simulink model "OFDMTxRx2211221"  (R2017b)
settings: Solver=VariableStepAuto  StartTime=0.0  StopTime=10  RelTol=1e-3
InitFcn:
  | Ts = 1e-6;
  | simParams.Ts = Ts;
  | simParams.TsTx = Ts;
  | simParams.TsRx = Ts;
  | simParams.nFFT = 1024;
  | simParams.lengthCP = 128;
  | nFFT = simParams.nFFT;
  | simParams.NSubcarriers = 398;
  | simParams.windowing = 16;
undefined symbols (not defined in the file): fft_size, i
libraries: hdlsllib x35, simulink x28, simulink_need_slupdate x17, dspmathops x5, dspxfrm3 x3, dspsigops x2, commdigbbndam3 x1, commrflib2 x1, commseqgen3 x1
(part 2 of 3)

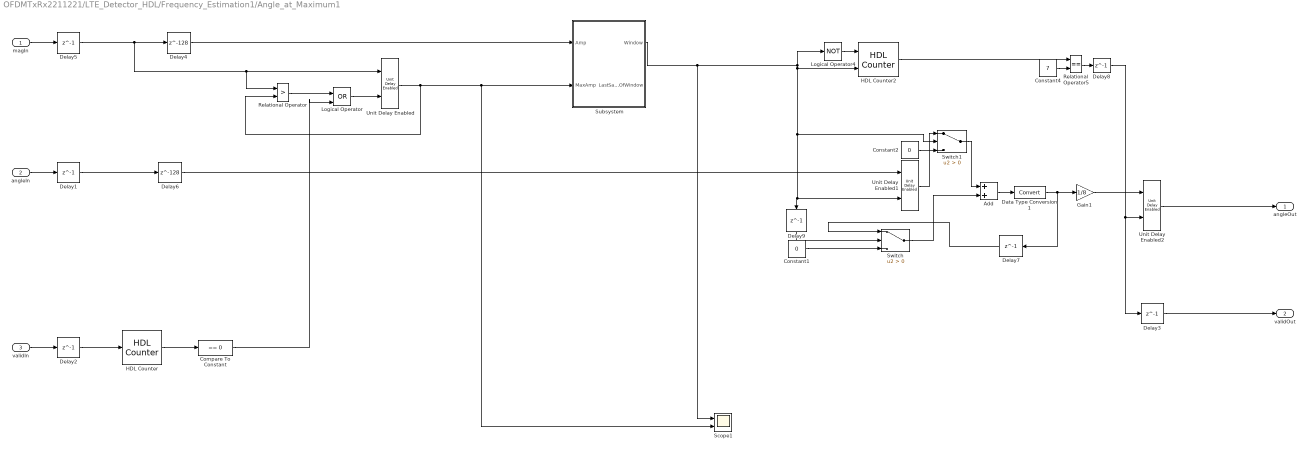
== system OFDMTxRx2211221/LTE_Detector_HDL/Frequency_Estimation1/Angle_at_Maximum1 ==
  magIn : Inport
  angleIn : Inport  Port=2
  validIn : Inport  Port=3
  Add : Sum
  Compare To Constant : simulink/Logic and Bit Operations/Compare To Constant  relop===  const=0  OutDataTypeStr=boolean
  Constant1 : Constant  Value=0
  Constant2 : Constant  Value=0
  Constant4 : Constant  Value=7
  Data Type Conversion1 : DataTypeConversion
  Delay{1..3,5,7..9} (7 alike) : Delay  DelayLength=1  InitialCondition=0  UseCircularBuffer=on
  Delay4 : Delay  DelayLength=128  InitialCondition=0  UseCircularBuffer=on
  Delay6 : Delay  DelayLength=128  InitialCondition=0  UseCircularBuffer=on
  Gain1 : Gain  Gain=1/8
  HDL Counter : hdlsllib/Sources/HDL Counter  CountType=Count limited  CountInit=0  CountStep=1  CountMax=1152  CountFromType=Initial value  CountFrom=0  CountResetPort=off  CountLoadPort=off  CountEnbPort=on  CountDirPort=off  CountDataType=Unsigned  CountWordLen=11  CountFracLen=0  CountSampTime=1
      settings: SourceProductBaseCode=HD
  HDL Counter2 : hdlsllib/Sources/HDL Counter  CountType=Count limited  CountInit=0  CountStep=1  CountMax=7  CountFromType=Initial value  CountFrom=0  CountResetPort=on  CountLoadPort=off  CountEnbPort=on  CountDirPort=off  CountDataType=Unsigned  CountWordLen=3  CountFracLen=0  CountSampTime=1
      settings: SourceProductBaseCode=HD
  Logical Operator : Logic  Operator=OR  IconShape=distinctive  AllPortsSameDT=off  OutDataTypeStr=boolean
  Logical Operator4 : Logic  Operator=NOT  IconShape=distinctive  AllPortsSameDT=off  OutDataTypeStr=boolean
  Relational Operator : RelationalOperator  Operator=>  OutDataTypeStr=boolean  RndMeth=Nearest
  Relational Operator5 : RelationalOperator  Operator===  OutDataTypeStr=boolean  RndMeth=Nearest
  Scope1 : Scope  NumInputPorts=2
  Subsystem : Subsystem
  Switch : Switch  Criteria=u2 > Threshold
  Switch1 : Switch  Criteria=u2 > Threshold
  Unit Delay Enabled : simulink_need_slupdate/Unit Delay Enabled  vinit=0.0  tsamp=-1
      settings: SourceProductName=Simulink  SourceProductBaseCode=SL
  Unit Delay Enabled1 : simulink_need_slupdate/Unit Delay Enabled  vinit=0.0  tsamp=-1
      settings: SourceProductName=Simulink  SourceProductBaseCode=SL
  Unit Delay Enabled2 : simulink_need_slupdate/Unit Delay Enabled  vinit=0.0  tsamp=-1
      settings: SourceProductName=Simulink  SourceProductBaseCode=SL
  angleOut : Outport
  validOut : Outport  Port=2
  wires:
  Delay4/1 -> Subsystem/1(Amp)
  Unit Delay Enabled1/1 -> Switch1/1
  Unit Delay Enabled2/1 -> angleOut/1
  Compare To Constant/1 -> Logical Operator/2
  Logical Operator/1 -> Unit Delay Enabled/2
  Constant1/1 -> Switch/3
  Delay7/1 -> Switch/1
  Delay3/1 -> validOut/1
  Constant2/1 -> Switch1/3
  Gain1/1 -> Unit Delay Enabled2/1
  Subsystem/1(Window) -> Scope1/1, Switch1/2, Delay9/1, Unit Delay Enabled1/2, HDL Counter2/2, Logical Operator4/1
  Delay9/1 -> Switch/2
  Unit Delay Enabled/1 -> Scope1/2, Subsystem/2(MaxAmp), Relational Operator/2
  Data Type Conversion1/1 -> Delay7/1, Gain1/1
  Logical Operator4/1 -> HDL Counter2/1
  Switch1/1 -> Add/1
  Add/1 -> Data Type Conversion1/1
  Relational Operator5/1 -> Delay8/1
  Delay2/1 -> HDL Counter/1
  HDL Counter2/1 -> Relational Operator5/1
  Constant4/1 -> Relational Operator5/2
  Delay8/1 -> Unit Delay Enabled2/2, Delay3/1
  Delay6/1 -> Unit Delay Enabled1/1
  Delay5/1 -> Relational Operator/1, Unit Delay Enabled/1, Delay4/1
  Delay1/1 -> Delay6/1
  validIn/1 -> Delay2/1
  Relational Operator/1 -> Logical Operator/1
  angleIn/1 -> Delay1/1
  HDL Counter/1 -> Compare To Constant/1
  magIn/1 -> Delay5/1
  Switch/1 -> Add/2

== system OFDMTxRx2211221/LTE_Detector_HDL/Frequency_Estimation1/Cyclic_Prefix_Correlator ==
  dataIn : Inport
  Delay1 : Delay  DelayLength=1  InitialCondition=0  UseCircularBuffer=on
  Delay2 : Delay  DelayLength=1024  InitialCondition=0
  Delay3 : Delay  DelayLength=1  InitialCondition=0  UseCircularBuffer=on
  Delay5 : Delay  DelayLength=1  InitialCondition=0  UseCircularBuffer=on
  Moving_Average : Subsystem
  Product : Product  OutDataTypeStr=fixdt(1,24,23)  RndMeth=Round
  Slot_Average : Subsystem
  complexConj : Math  Operator=conj  SaturateOnIntegerOverflow=on
  corrOut : Outport
  wires:
  Delay3/1 -> Product/2
  Delay2/1 -> complexConj/1
  complexConj/1 -> Delay3/1
  Delay1/1 -> Product/1
  Delay5/1 -> Moving_Average/1(dataIn)
  dataIn/1 -> Delay2/1, Delay1/1
  Product/1 -> Delay5/1
  Moving_Average/1(dataOut) -> Slot_Average/1(dataIn)
  Slot_Average/1(dataOut) -> corrOut/1

== system OFDMTxRx2211221/LTE_Detector_HDL/Frequency_Estimation1/Rect_to_Polar ==
  dataIn : Inport
  Complex to Magnitude-Angle HDL Optimized : dspmathops/Complex to Magnitude-Angle HDL Optimized  NumIterationsSource=Auto  NumIterations=16  OutputFormat=Magnitude and angle  AngleFormat=Normalized  ScaleOutput=on  SimulateUsing=Code generation
      settings: SourceProductName=DSP System Toolbox  SourceProductBaseCode=DS
  Constant : Constant  OutDataTypeStr=boolean  SampleTime=simParams.TsRx
  Delay1 : Delay  InitialCondition=0  UseCircularBuffer=on
  Delay2 : Delay  DelayLength=1  InitialCondition=0  UseCircularBuffer=on
  Delay3 : Delay  DelayLength=1  InitialCondition=0  UseCircularBuffer=on
  Delay4 : Delay  DelayLength=1  InitialCondition=0  UseCircularBuffer=on
  Delay5 : Delay  InitialCondition=0  UseCircularBuffer=on
  Gain : Gain  Gain=0.5  OutDataTypeStr=fixdt(1,27,27)
  Signal Specification1 : SignalSpecification  Dimensions=1
  magOut : Outport
  angleOut : Outport  Port=2
  validOut : Outport  Port=3
  wires:
  Gain/1 -> angleOut/1
  dataIn/1 -> Signal Specification1/1
  Constant/1 -> Delay1/1
  Delay5/1 -> Complex to Magnitude-Angle HDL Optimized/1
  Delay1/1 -> Complex to Magnitude-Angle HDL Optimized/2
  Delay2/1 -> magOut/1
  Delay3/1 -> Gain/1
  Delay4/1 -> validOut/1
  Complex to Magnitude-Angle HDL Optimized/1 -> Delay2/1
  Complex to Magnitude-Angle HDL Optimized/3 -> Delay4/1
  Complex to Magnitude-Angle HDL Optimized/2 -> Delay3/1
  Signal Specification1/1 -> Delay5/1

== system OFDMTxRx2211221/LTE_Detector_HDL/Frequency_Estimation2/Angle_at_Maximum ==
  note: This subsystem records the maximum CP correlation level, and the corresponding phase angle of the result, across windows of time equivalent to 1 slot (960 samples). A counter is used to reset the running max and record the final phase value, which is then passed to the output and qualified by the validOut signal.
  note: Store current mag & angle if mag is greater than previous max mag.
  note: This register stores the current running max magnitude in the current time window
  magIn : Inport
  angleIn : Inport  Port=2
  validIn : Inport  Port=3
  Compare To Constant : simulink/Logic and Bit Operations/Compare To Constant  relop===  const=0  OutDataTypeStr=boolean
  Delay{1..3,5} (4 alike) : Delay  DelayLength=1  InitialCondition=0  UseCircularBuffer=on
  HDL Counter : hdlsllib/Sources/HDL Counter  CountType=Count limited  CountInit=0  CountStep=1  CountMax=1152  CountFromType=Initial value  CountFrom=0  CountResetPort=off  CountLoadPort=off  CountEnbPort=on  CountDirPort=off  CountDataType=Unsigned  CountWordLen=11  CountFracLen=0  CountSampTime=1
      settings: SourceProductBaseCode=HD
  Logical Operator : Logic  Operator=OR  IconShape=distinctive  AllPortsSameDT=off  OutDataTypeStr=boolean
  Relational Operator : RelationalOperator  Operator=>  OutDataTypeStr=boolean  RndMeth=Nearest
  Unit Delay Enabled : simulink_need_slupdate/Unit Delay Enabled  vinit=0.0  tsamp=-1
      settings: SourceProductName=Simulink  SourceProductBaseCode=SL
  Unit Delay Enabled1 : simulink_need_slupdate/Unit Delay Enabled  vinit=0.0  tsamp=-1
      settings: SourceProductName=Simulink  SourceProductBaseCode=SL
  Unit Delay Enabled2 : simulink_need_slupdate/Unit Delay Enabled  vinit=0.0  tsamp=-1
      settings: SourceProductName=Simulink  SourceProductBaseCode=SL
  angleOut : Outport
  validOut : Outport  Port=2
  wires:
  magIn/1 -> Delay5/1
  angleIn/1 -> Delay1/1
  HDL Counter/1 -> Compare To Constant/1
  Compare To Constant/1 -> Unit Delay Enabled2/2, Logical Operator/2, Delay3/1
  Unit Delay Enabled1/1 -> Unit Delay Enabled2/1
  validIn/1 -> Delay2/1
  Delay5/1 -> Relational Operator/1, Unit Delay Enabled/1
  Delay2/1 -> HDL Counter/1
  Unit Delay Enabled2/1 -> angleOut/1
  Delay3/1 -> validOut/1
  Unit Delay Enabled/1 -> Relational Operator/2
  Relational Operator/1 -> Logical Operator/1
  Logical Operator/1 -> Unit Delay Enabled1/2, Unit Delay Enabled/2
  Delay1/1 -> Unit Delay Enabled1/1

== system OFDMTxRx2211221/LTE_Detector_HDL/Frequency_Estimation2/Cyclic_Prefix_Correlator ==
  note: Correlate the signal with itself
      | delayed by the FFT length (128 samples).
  note: Integrate across part of the CP length, which is 9 samples. However we use 8 samples here to optimize for HDL implementation.
  note: Finally average across 7 OFDM symbols, i.e. the number in
      | each slot.
  dataIn : Inport
  Delay1 : Delay  DelayLength=1  InitialCondition=0  UseCircularBuffer=on
  Delay2 : Delay  DelayLength=1024  InitialCondition=0
  Delay3 : Delay  DelayLength=1  InitialCondition=0  UseCircularBuffer=on
  Delay5 : Delay  DelayLength=1  InitialCondition=0  UseCircularBuffer=on
  Moving_Average : Subsystem
  Product : Product  OutDataTypeStr=fixdt(1,24,23)  RndMeth=Round
  Slot_Average : Subsystem
  complexConj : Math  Operator=conj  SaturateOnIntegerOverflow=on
  corrOut : Outport
  wires:
  Product/1 -> Delay5/1
  Delay3/1 -> Product/2
  Delay2/1 -> complexConj/1
  Slot_Average/1(dataOut) -> corrOut/1
  Moving_Average/1(dataOut) -> Slot_Average/1(dataIn)
  complexConj/1 -> Delay3/1
  Delay5/1 -> Moving_Average/1(dataIn)
  Delay1/1 -> Product/1
  dataIn/1 -> Delay2/1, Delay1/1

== system OFDMTxRx2211221/LTE_Detector_HDL/Frequency_Estimation2/Rect_to_Polar ==
  dataIn : Inport
  Complex to Magnitude-Angle HDL Optimized : dspmathops/Complex to Magnitude-Angle HDL Optimized  NumIterationsSource=Auto  NumIterations=16  OutputFormat=Magnitude and angle  AngleFormat=Normalized  ScaleOutput=on  SimulateUsing=Code generation
      settings: SourceProductName=DSP System Toolbox  SourceProductBaseCode=DS
  Constant : Constant  OutDataTypeStr=boolean  SampleTime=simParams.TsRx
  Delay1 : Delay  InitialCondition=0  UseCircularBuffer=on
  Delay2 : Delay  DelayLength=1  InitialCondition=0  UseCircularBuffer=on
  Delay3 : Delay  DelayLength=1  InitialCondition=0  UseCircularBuffer=on
  Delay4 : Delay  DelayLength=1  InitialCondition=0  UseCircularBuffer=on
  Delay5 : Delay  InitialCondition=0  UseCircularBuffer=on
  Gain : Gain  Gain=0.5  OutDataTypeStr=fixdt(1,27,27)
  Signal Specification1 : SignalSpecification  Dimensions=1
  magOut : Outport
  angleOut : Outport  Port=2
  validOut : Outport  Port=3
  wires:
  Gain/1 -> angleOut/1
  dataIn/1 -> Signal Specification1/1
  Constant/1 -> Delay1/1
  Delay5/1 -> Complex to Magnitude-Angle HDL Optimized/1
  Delay1/1 -> Complex to Magnitude-Angle HDL Optimized/2
  Delay2/1 -> magOut/1
  Delay3/1 -> Gain/1
  Delay4/1 -> validOut/1
  Complex to Magnitude-Angle HDL Optimized/1 -> Delay2/1
  Complex to Magnitude-Angle HDL Optimized/3 -> Delay4/1
  Complex to Magnitude-Angle HDL Optimized/2 -> Delay3/1
  Signal Specification1/1 -> Delay5/1

== system OFDMTxRx2211221/LTE_Detector_HDL/Переформирование отсчетов/Rect_to_Polar ==
  dataIn : Inport
  "ValidIn " : Inport  Port=2
  Complex to Magnitude-Angle HDL Optimized : dspmathops/Complex to Magnitude-Angle HDL Optimized  NumIterationsSource=Auto  NumIterations=16  OutputFormat=Magnitude and angle  AngleFormat=Normalized  ScaleOutput=on  SimulateUsing=Code generation
      settings: SourceProductName=DSP System Toolbox  SourceProductBaseCode=DS
  Delay1 : Delay  InitialCondition=0  UseCircularBuffer=on
  Delay2 : Delay  DelayLength=1  InitialCondition=0  UseCircularBuffer=on
  Delay3 : Delay  DelayLength=1  InitialCondition=0  UseCircularBuffer=on
  Delay4 : Delay  DelayLength=1  InitialCondition=0  UseCircularBuffer=on
  Delay5 : Delay  InitialCondition=0  UseCircularBuffer=on
  Signal Specification1 : SignalSpecification  Dimensions=1
  magOut : Outport
  angleOut : Outport  Port=2
  validOut : Outport  Port=3
  wires:
  Delay3/1 -> angleOut/1
  dataIn/1 -> Signal Specification1/1
  "ValidIn "/1 -> Delay1/1
  Delay5/1 -> Complex to Magnitude-Angle HDL Optimized/1
  Delay1/1 -> Complex to Magnitude-Angle HDL Optimized/2
  Delay2/1 -> magOut/1
  Delay4/1 -> validOut/1
  Complex to Magnitude-Angle HDL Optimized/1 -> Delay2/1
  Complex to Magnitude-Angle HDL Optimized/3 -> Delay4/1
  Complex to Magnitude-Angle HDL Optimized/2 -> Delay3/1
  Signal Specification1/1 -> Delay5/1

== system OFDMTxRx2211221/LTE_Detector_HDL/Подстройка по фазе/Подкрутка фазы ==
  PureSig : Inport
  "DifPhase " : Inport  Port=2
  Constant1 : Constant  Value=3.14159265359  SampleTime=simParams.Ts
  Constant13 : Constant  Value=complex(0-i)  SampleTime=simParams.Ts
  Pow1 : Math  RndMeth=Zero  SaturateOnIntegerOverflow=on
  Product3 : Product  Inputs=3
  Product4 : Product
  Out1 : Outport
  wires:
  PureSig/1 -> Product4/1
  Product4/1 -> Out1/1
  Product3/1 -> Pow1/1
  Constant13/1 -> Product3/2
  Pow1/1 -> Product4/2
  "DifPhase "/1 -> Product3/1
  Constant1/1 -> Product3/3

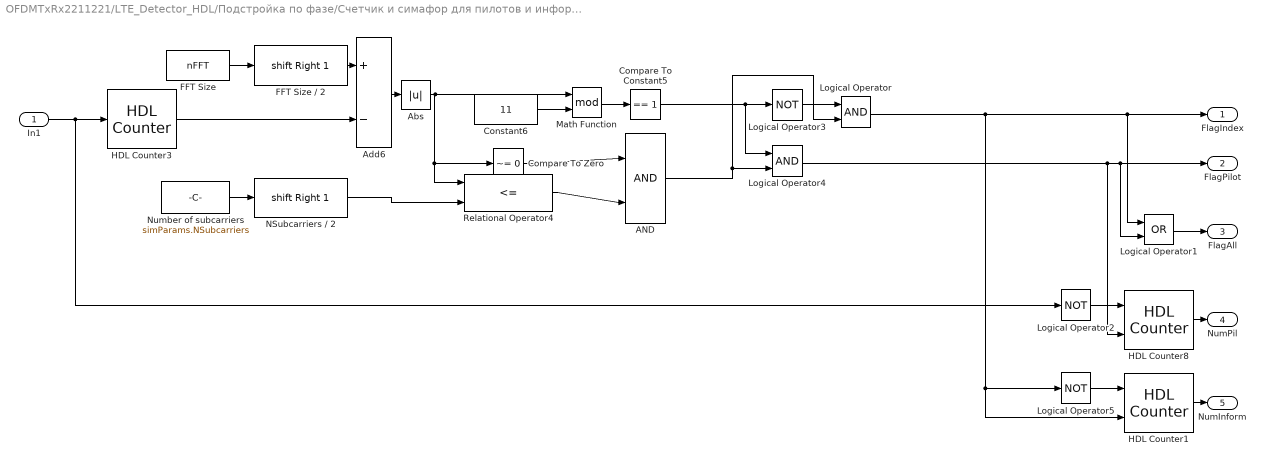
== system OFDMTxRx2211221/LTE_Detector_HDL/Подстройка по фазе/Счетчик и симафор для пилотов и информационных ==
  In1 : Inport
  AND : Logic  IconShape=distinctive  AllPortsSameDT=off  OutDataTypeStr=boolean
  Abs : Abs
  Add6 : Sum  Inputs=+-  OutDataTypeStr=fixdt(1,16,0)
  Compare To Constant5 : simulink/Logic and Bit Operations/Compare To Constant  relop===  const=1  OutDataTypeStr=boolean
  Compare To Zero : simulink/Logic and Bit Operations/Compare To Zero  relop=~=  OutDataTypeStr=boolean
  Constant6 : Constant  Value=11  OutDataTypeStr=int16  SampleTime=simParams.Ts
  FFT Size : Constant  Value=nFFT  OutDataTypeStr=fixdt(0,ceil(log2(simParams.nFFT))+1,0)  SampleTime=Ts
  FFT Size / 2 : ArithShift  BitShiftNumber=1  BitShiftDirection=Right
  HDL Counter1 : hdlsllib/Sources/HDL Counter  CountType=Count limited  CountInit=0  CountStep=1  CountMax=80  CountFromType=Initial value  CountFrom=0  CountResetPort=on  CountLoadPort=off  CountEnbPort=on  CountDirPort=off  CountDataType=Unsigned  CountWordLen=8  CountFracLen=0  CountSampTime=1
      settings: SourceProductBaseCode=HD
  HDL Counter3 : hdlsllib/Sources/HDL Counter  CountType=Count limited  CountInit=0  CountStep=1  CountMax=1023  CountFromType=Initial value  CountFrom=0  CountResetPort=off  CountLoadPort=off  CountEnbPort=on  CountDirPort=off  CountDataType=Unsigned  CountWordLen=11  CountFracLen=0  CountSampTime=1
      settings: SourceProductBaseCode=HD
  HDL Counter8 : hdlsllib/Sources/HDL Counter  CountType=Count limited  CountInit=0  CountStep=1  CountMax=80  CountFromType=Initial value  CountFrom=0  CountResetPort=on  CountLoadPort=off  CountEnbPort=on  CountDirPort=off  CountDataType=Unsigned  CountWordLen=8  CountFracLen=0  CountSampTime=1
      settings: SourceProductBaseCode=HD
  Logical Operator : Logic  AllPortsSameDT=off  OutDataTypeStr=boolean
  Logical Operator1 : Logic  Operator=OR  AllPortsSameDT=off  OutDataTypeStr=boolean
  Logical Operator2 : Logic  Operator=NOT  Inputs=1  AllPortsSameDT=off  OutDataTypeStr=boolean
  Logical Operator3 : Logic  Operator=NOT  Inputs=1  AllPortsSameDT=off  OutDataTypeStr=boolean
  Logical Operator4 : Logic  AllPortsSameDT=off  OutDataTypeStr=boolean
  Logical Operator5 : Logic  Operator=NOT  Inputs=1  AllPortsSameDT=off  OutDataTypeStr=boolean
  Math Function : Math  Operator=mod  RndMeth=Zero  SaturateOnIntegerOverflow=on
  NSubcarriers / 2 : ArithShift  BitShiftNumber=1  BitShiftDirection=Right
  Number of subcarriers : Constant  Value=simParams.NSubcarriers  OutDataTypeStr=fixdt(0,12,0)  SampleTime=Ts
  Relational Operator4 : RelationalOperator  Operator=<=  OutDataTypeStr=boolean  RndMeth=Nearest
  FlagIndex : Outport
  FlagPilot : Outport  Port=2
  FlagAll : Outport  Port=3
  NumPil : Outport  Port=4
  NumInform : Outport  Port=5
  wires:
  In1/1 -> Logical Operator2/1, HDL Counter3/1
  HDL Counter3/1 -> Add6/2
  FFT Size/1 -> FFT Size / 2/1
  Logical Operator/1 -> HDL Counter1/2, Logical Operator5/1, Logical Operator1/1, FlagIndex/1
  Constant6/1 -> Math Function/2
  AND/1 -> Logical Operator4/2, Logical Operator/2
  Number of subcarriers/1 -> NSubcarriers / 2/1
  Add6/1 -> Abs/1
  Logical Operator3/1 -> Logical Operator/1
  Abs/1 -> Relational Operator4/1, Compare To Zero/1, Math Function/1
  NSubcarriers / 2/1 -> Relational Operator4/2
  FFT Size / 2/1 -> Add6/1
  Compare To Zero/1 -> AND/1
  Math Function/1 -> Compare To Constant5/1
  Relational Operator4/1 -> AND/2
  Logical Operator4/1 -> HDL Counter8/2, Logical Operator1/2, FlagPilot/1
  Compare To Constant5/1 -> Logical Operator4/1, Logical Operator3/1
  Logical Operator1/1 -> FlagAll/1
  Logical Operator2/1 -> HDL Counter8/1
  HDL Counter8/1 -> NumPil/1
  Logical Operator5/1 -> HDL Counter1/1
  HDL Counter1/1 -> NumInform/1

== system OFDMTxRx2211221/LTE_Detector_HDL/Подстройка по фазе/Устранение 2pi неопределенности и вычисление разности фаз1 ==
  "Фаза \"левого\" пилота" : Inport
  "Фаза \"правого\" пилота" : Inport  Port=2
  Add8 : Sum  Inputs=+-
  Add9 : Sum  Inputs=-+
  Constant8 : Constant  Value=2  OutDataTypeStr=double  SampleTime=simParams.Ts
  Relational Operator7 : RelationalOperator  Operator=>  OutDataTypeStr=boolean  RndMeth=Nearest
  Switch10 : Switch  Criteria=u2 ~= 0
  "Разность фаз " : Outport
  wires:
  Switch10/1 -> Add9/2
  Add8/1 -> Switch10/1
  "Фаза \"правого\" пилота"/1 -> Switch10/3, Relational Operator7/1, Add8/1
  Constant8/1 -> Add8/2
  "Фаза \"левого\" пилота"/1 -> Add9/1, Relational Operator7/2
  Relational Operator7/1 -> Switch10/2
  Add9/1 -> "Разность фаз "/1

== system OFDMTxRx2211221/LTE_Detector_HDL/Эквалайзинг забита только формула/Subsystem ==
  In1 : Inport
  2interp : Subsystem
  Constant1 : Constant  Value=3
  Delay1 : Delay  DelayLength=11  InitialCondition=0  UseCircularBuffer=on
  Delay6 : Delay  DelayLength=21  InitialCondition=0  UseCircularBuffer=on
  Divide2 : Product  Inputs=*/  SaturateOnIntegerOverflow=on  RndMeth=Zero
  Out1 : Outport
  Out2 : Outport  Port=2
  Out3 : Outport  Port=3
  wires:
  2interp/3(c) -> Out3/1
  Delay1/1 -> 2interp/2(y2)
  Delay6/1 -> 2interp/1(y1)
  In1/1 -> Divide2/2
  2interp/1(a) -> Out1/1
  2interp/2(b) -> Out2/1
  Constant1/1 -> Divide2/1
  Divide2/1 -> 2interp/3(y3), Delay6/1, Delay1/1

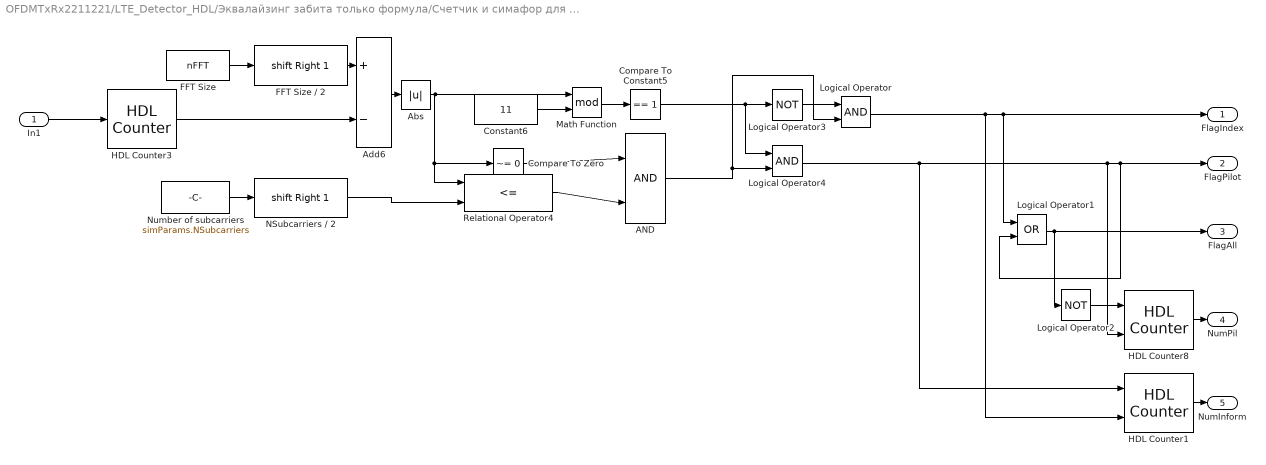
== system OFDMTxRx2211221/LTE_Detector_HDL/Эквалайзинг забита только формула/Счетчик и симафор для пилотов и информационных ==
  In1 : Inport
  AND : Logic  IconShape=distinctive  AllPortsSameDT=off  OutDataTypeStr=boolean
  Abs : Abs
  Add6 : Sum  Inputs=+-  OutDataTypeStr=fixdt(1,16,0)
  Compare To Constant5 : simulink/Logic and Bit Operations/Compare To Constant  relop===  const=1  OutDataTypeStr=boolean
  Compare To Zero : simulink/Logic and Bit Operations/Compare To Zero  relop=~=  OutDataTypeStr=boolean
  Constant6 : Constant  Value=11  OutDataTypeStr=int16  SampleTime=simParams.Ts
  FFT Size : Constant  Value=nFFT  OutDataTypeStr=fixdt(0,ceil(log2(simParams.nFFT))+1,0)  SampleTime=Ts
  FFT Size / 2 : ArithShift  BitShiftNumber=1  BitShiftDirection=Right
  HDL Counter1 : hdlsllib/Sources/HDL Counter  CountType=Count limited  CountInit=0  CountStep=1  CountMax=80  CountFromType=Initial value  CountFrom=0  CountResetPort=on  CountLoadPort=off  CountEnbPort=on  CountDirPort=off  CountDataType=Unsigned  CountWordLen=8  CountFracLen=0  CountSampTime=1
      settings: SourceProductBaseCode=HD
  HDL Counter3 : hdlsllib/Sources/HDL Counter  CountType=Count limited  CountInit=0  CountStep=1  CountMax=1023  CountFromType=Initial value  CountFrom=0  CountResetPort=off  CountLoadPort=off  CountEnbPort=on  CountDirPort=off  CountDataType=Unsigned  CountWordLen=11  CountFracLen=0  CountSampTime=1
      settings: SourceProductBaseCode=HD
  HDL Counter8 : hdlsllib/Sources/HDL Counter  CountType=Count limited  CountInit=0  CountStep=1  CountMax=80  CountFromType=Initial value  CountFrom=0  CountResetPort=on  CountLoadPort=off  CountEnbPort=on  CountDirPort=off  CountDataType=Unsigned  CountWordLen=8  CountFracLen=0  CountSampTime=1
      settings: SourceProductBaseCode=HD
  Logical Operator : Logic  AllPortsSameDT=off  OutDataTypeStr=boolean
  Logical Operator1 : Logic  Operator=OR  AllPortsSameDT=off  OutDataTypeStr=boolean
  Logical Operator2 : Logic  Operator=NOT  Inputs=1  AllPortsSameDT=off  OutDataTypeStr=boolean
  Logical Operator3 : Logic  Operator=NOT  Inputs=1  AllPortsSameDT=off  OutDataTypeStr=boolean
  Logical Operator4 : Logic  AllPortsSameDT=off  OutDataTypeStr=boolean
  Math Function : Math  Operator=mod  RndMeth=Zero  SaturateOnIntegerOverflow=on
  NSubcarriers / 2 : ArithShift  BitShiftNumber=1  BitShiftDirection=Right
  Number of subcarriers : Constant  Value=simParams.NSubcarriers  OutDataTypeStr=fixdt(0,12,0)  SampleTime=Ts
  Relational Operator4 : RelationalOperator  Operator=<=  OutDataTypeStr=boolean  RndMeth=Nearest
  FlagIndex : Outport
  FlagPilot : Outport  Port=2
  FlagAll : Outport  Port=3
  NumPil : Outport  Port=4
  NumInform : Outport  Port=5
  wires:
  In1/1 -> HDL Counter3/1
  HDL Counter3/1 -> Add6/2
  FFT Size/1 -> FFT Size / 2/1
  Logical Operator/1 -> HDL Counter1/2, FlagIndex/1, Logical Operator1/1
  Constant6/1 -> Math Function/2
  AND/1 -> Logical Operator4/2, Logical Operator/2
  Number of subcarriers/1 -> NSubcarriers / 2/1
  Add6/1 -> Abs/1
  Logical Operator3/1 -> Logical Operator/1
  Abs/1 -> Relational Operator4/1, Compare To Zero/1, Math Function/1
  NSubcarriers / 2/1 -> Relational Operator4/2
  FFT Size / 2/1 -> Add6/1
  Compare To Zero/1 -> AND/1
  Math Function/1 -> Compare To Constant5/1
  Relational Operator4/1 -> AND/2
  Compare To Constant5/1 -> Logical Operator4/1, Logical Operator3/1
  Logical Operator1/1 -> Logical Operator2/1, FlagAll/1
  Logical Operator2/1 -> HDL Counter8/1
  HDL Counter8/1 -> NumPil/1
  Logical Operator4/1 -> HDL Counter1/1, HDL Counter8/2, Logical Operator1/2, FlagPilot/1
  HDL Counter1/1 -> NumInform/1

== system OFDMTxRx2211221/DUT/symmetric /Add CP and windowing/FFT ==
  note: Set input of FFT to input wordlength + FFT growth to allow
      | the output of the FFT to scale. Maximum bit growth is equal
      | to log2(nFFT).
  dataIn : Inport
  validIn : Inport  Port=2
  Data Type Conversion : DataTypeConversion  OutDataTypeStr=fixdt(1,18,10)  RndMeth=Round
  Delay{1..2,4..5} (4 alike) : Delay  DelayLength=1  InitialCondition=0  InputProcessing=Columns as channels (frame based)
  FFT HDL Optimized : dspxfrm3/FFT HDL Optimized  FFTLength=1024  Architecture=Streaming Radix 2^2  ComplexMultiplication=Use 3 multipliers and 5 adders  BitReversedOutput=off  BitReversedInput=off  Normalize=off  SimulateUsing=Code generation  RoundingMethod=Floor  ResetInputPort=off  StartOutputPort=off  EndOutputPort=off
      settings: SourceProductName=DSP System Toolbox  SourceProductBaseCode=DS
  Signal Specification : SignalSpecification  Dimensions=1
  Signal Specification1 : SignalSpecification  Dimensions=1
  dataOut : Outport
  validOut : Outport  Port=2
  wires:
  Signal Specification1/1 -> FFT HDL Optimized/2
  Signal Specification/1 -> FFT HDL Optimized/1
  FFT HDL Optimized/2 -> Delay5/1
  FFT HDL Optimized/1 -> Delay4/1
  Delay4/1 -> Data Type Conversion/1
  Delay2/1 -> Signal Specification1/1
  dataIn/1 -> Delay1/1
  validIn/1 -> Delay2/1
  Delay1/1 -> Signal Specification/1
  Data Type Conversion/1 -> dataOut/1
  Delay5/1 -> validOut/1

== system OFDMTxRx2211221/DUT/symmetric /fORM1/Counter  ==
  note: Возможность переключать длину
      | циклического префикса для
      | обозначения начала кадра.
      | Пока что выключена. Идет 1024 +128 отсчетов.
  note: Счетчик символов в кадре
  note: Reset signal takes one clock cycle to register.
      | So reset should be triggered when count value
      | equals nFFT+CPlength-1 .
      | Hence use of nFFT-1.
  note: Первые отсчеты <0 и зарезервированы для Префикса.Посылается значение 1024.
      | После этого бины считаются 0->Nfft
  Add : Sum
  Compare To Zero : simulink/Logic and Bit Operations/Compare To Zero  relop===  OutDataTypeStr=boolean
  Compare To Zero1 : simulink/Logic and Bit Operations/Compare To Zero  relop=>=  OutDataTypeStr=boolean
  FFT Size : Constant  Value=simParams.nFFT-1  OutDataTypeStr=fixdt(0,ceil(log2(simParams.nFFT)),0)  SampleTime=simParams.Ts
  FFT Size1 : Constant  Value=simParams.nFFT  OutDataTypeStr=fixdt(0,ceil(log2(simParams.nFFT))+2,0)  SampleTime=simParams.Ts
  HDL Counter : hdlsllib/Sources/HDL Counter  CountType=Count limited  CountInit=0  CountStep=1  CountMax=6  CountFromType=Initial value  CountFrom=0  CountResetPort=off  CountLoadPort=off  CountEnbPort=on  CountDirPort=off  CountDataType=Unsigned  CountWordLen=3  CountFracLen=0  CountSampTime=1
      settings: SourceProductBaseCode=HD
  HDL Counter2 : hdlsllib/Sources/HDL Counter  CountType=Free running  CountInit=0  CountStep=1  CountMax=6  CountFromType=Initial value  CountFrom=0  CountResetPort=on  CountLoadPort=off  CountEnbPort=off  CountDirPort=off  CountDataType=Unsigned  CountWordLen=ceil(log2(simParams.nFFT))+1  CountFracLen=0  CountSampTime=1
      settings: SourceProductBaseCode=HD
  Length of first CP : Constant  Value=simParams.lengthCP  OutDataTypeStr=fixdt(0,ceil(log2(simParams.nFFT)),0)  SampleTime=simParams.Ts
  Length of other CPs : Constant  Value=simParams.lengthCP  OutDataTypeStr=fixdt(0,ceil(log2(simParams.nFFT)),0)  SampleTime=simParams.Ts
  Relational Operator : RelationalOperator  Operator===  OutDataTypeStr=boolean  RndMeth=Nearest
  Subtract : Sum  Inputs=+-  OutDataTypeStr=fixdt(1,ceil(log2(simParams.nFFT))+2,0)
  Switch : Switch  Criteria=u2 ~= 0
  Switch1 : Switch  Criteria=u2 ~= 0
  IFFT subcarrier : Outport
  wires:
  FFT Size/1 -> Add/1
  HDL Counter2/1 -> Subtract/1, Relational Operator/1  "Count"
  Switch/1 -> Subtract/2, Add/2
  Subtract/1 -> Compare To Zero1/1, Switch1/1
  HDL Counter/1 -> Compare To Zero/1
  FFT Size1/1 -> Switch1/3
  Compare To Zero/1 -> Switch/2
  Length of first CP/1 -> Switch/1
  [INCREMENT_SYMBOL] -> HDL Counter/1
  Switch1/1 -> IFFT subcarrier/1
  Add/1 -> Relational Operator/2
  Compare To Zero1/1 -> Switch1/2
  Length of other CPs/1 -> Switch/3
  Relational Operator/1 -> HDL Counter2/1, [INCREMENT_SYMBOL]

== system OFDMTxRx2211221/DUT/symmetric /fORM1/Rect_to_Polar ==
  dataIn : Inport
  dataIn1 : Inport  Port=2
  Complex to Magnitude-Angle HDL Optimized : dspmathops/Complex to Magnitude-Angle HDL Optimized  NumIterationsSource=Auto  NumIterations=16  OutputFormat=Magnitude and angle  AngleFormat=Radians  ScaleOutput=on  SimulateUsing=Code generation
      settings: SourceProductName=DSP System Toolbox  SourceProductBaseCode=DS
  Delay1 : Delay  InitialCondition=0  UseCircularBuffer=on
  Delay2 : Delay  DelayLength=1  InitialCondition=0  UseCircularBuffer=on
  Delay3 : Delay  DelayLength=1  InitialCondition=0  UseCircularBuffer=on
  Delay4 : Delay  DelayLength=1  InitialCondition=0  UseCircularBuffer=on
  Delay5 : Delay  InitialCondition=0  UseCircularBuffer=on
  Signal Specification1 : SignalSpecification  Dimensions=1
  magOut : Outport
  angleOut : Outport  Port=2
  validOut : Outport  Port=3
  wires:
  Delay3/1 -> angleOut/1
  dataIn/1 -> Signal Specification1/1
  dataIn1/1 -> Delay1/1
  Delay5/1 -> Complex to Magnitude-Angle HDL Optimized/1
  Delay1/1 -> Complex to Magnitude-Angle HDL Optimized/2
  Delay2/1 -> magOut/1
  Delay4/1 -> validOut/1
  Complex to Magnitude-Angle HDL Optimized/1 -> Delay2/1
  Complex to Magnitude-Angle HDL Optimized/3 -> Delay4/1
  Complex to Magnitude-Angle HDL Optimized/2 -> Delay3/1
  Signal Specification1/1 -> Delay5/1

== system OFDMTxRx2211221/DUT/symmetric /Сдвиг в симметричный вид /Compute_Read_Address ==
  note: XOR with FFT size/2 performs the fftshift on the address
      | as it flips the MSB of the index in the IFFT,
      | while XOR with FFT size flips the ping/pong
  note: select enough bits to represent 2*fft_size addresses
  note: Ping/Pong Read Address so reading from half of BlockRAM not being written to.
  note: Load Read Ptr with 0
      | and count up to fft_size  to read out data
  note: When rdEnable goes high toggle offset for Ping/Pong buffer for Read Ptr.
      | Make sure REAd and WRITE Ptr are not in same section of Ping/Pong
  note: Initial counter output is FFT size setting the counter enable to '0'.
      | When the rdEnable signal comes in, the value of 0 is loaded into
      | the counter accumulator AND output. This triggers the
      | enable signal to '1', and the counter will count up to FFT size
      | before the enable goes to '0', where the counter will remain until
      | the next load signal arrives.
  note: Alternates between outputting a '0' and '1'
      | each time the read signal is toggled high.
  rdEnable : Inport
  Bit Slice : hdlsllib/Logic and Bit Operations/Bit Slice  lidx=log2(simParams.nFFT)  ridx=0
  Bitwise Operator1 : simulink/Logic and Bit Operations/Bitwise Operator  logicop=XOR  UseBitMask=off  NumInputPorts=2  BitMask=fft_size/2  BitMaskRealWorld=Stored Integer
  Compare To Constant4 : simulink/Logic and Bit Operations/Compare To Constant  relop=<  const=simParams.nFFT  OutDataTypeStr=boolean
  Constant3 : Constant  Value=simParams.nFFT/2  OutDataTypeStr=uint16  SampleTime=simParams.TsTx
  Constant4 : Constant  Value=simParams.nFFT+simParams.nFFT/2  OutDataTypeStr=uint16  SampleTime=simParams.TsTx
  Constant6 : Constant  Value=0  OutDataTypeStr=uint16  SampleTime=simParams.TsTx
  Delay3 : Delay  DelayLength=1
  HDL Counter1 : hdlsllib/Sources/HDL Counter  CountType=Free running  CountInit=simParams.nFFT  CountStep=1  CountMax=10  CountFromType=Initial value  CountFrom=simParams.nFFT  CountResetPort=off  CountLoadPort=on  CountEnbPort=on  CountDirPort=off  CountDataType=Unsigned  CountWordLen=16  CountFracLen=0  CountSampTime=1
      settings: SourceProductBaseCode=HD
  Not : Logic  Operator=NOT  IconShape=distinctive  AllPortsSameDT=off  OutDataTypeStr=boolean
  Scope1 : Scope  NumInputPorts=2
  Switch : Switch  Criteria=u2 ~= 0  Threshold=384
  Switch2 : Switch  Criteria=u2 ~= 0  Threshold=384
  rdAddr : Outport
  rdValid : Outport  Port=2
  wires:
  HDL Counter1/1 -> Scope1/2, Compare To Constant4/1, Bitwise Operator1/1
  Compare To Constant4/1 -> HDL Counter1/3, rdValid/1
  Switch2/1 -> Delay3/1, Switch/2
  Delay3/1 -> Switch2/3, Not/1
  Not/1 -> Switch2/1
  Constant6/1 -> HDL Counter1/2
  rdEnable/1 -> Scope1/1, HDL Counter1/1, Switch2/2
  Bit Slice/1 -> rdAddr/1
  Constant4/1 -> Switch/3
  Constant3/1 -> Switch/1
  Switch/1 -> Bitwise Operator1/2
  Bitwise Operator1/1 -> Bit Slice/1

== system OFDMTxRx2211221/LTE_Detector_HDL/Frequency_Estimation/Angle_at_Maximum/Задержка максимального значения ==
  AmpIn : Inport
  "Reset " : Inport  Port=2
  Logical Operator : Logic  Operator=OR  IconShape=distinctive  AllPortsSameDT=off  OutDataTypeStr=boolean
  Relational Operator : RelationalOperator  Operator=>  OutDataTypeStr=boolean  RndMeth=Nearest
  Unit Delay Enabled : simulink_need_slupdate/Unit Delay Enabled  vinit=0.0  tsamp=-1
      settings: SourceProductName=Simulink  SourceProductBaseCode=SL
  "MagMax " : Outport
  wires:
  Logical Operator/1 -> Unit Delay Enabled/2
  Unit Delay Enabled/1 -> "MagMax "/1, Relational Operator/2
  Relational Operator/1 -> Logical Operator/1
  "Reset "/1 -> Logical Operator/2
  AmpIn/1 -> Relational Operator/1, Unit Delay Enabled/1

== system OFDMTxRx2211221/LTE_Detector_HDL/Frequency_Estimation/Angle_at_Maximum/Нахождение окрестности середины ЗИ ==
  note: Условие на превышение уровня 0.7 АКФ
  MagIn : Inport
  MagMax : Inport  Port=2
  "Reset " : Inport  Port=3
  Add : Sum
  Add1 : Sum  Inputs=+-
  Constant : Constant  Value=2*10^-4
  Constant3 : Constant  Value=4
  Delay1 : Delay  DelayLength=100  InitialCondition=0  UseCircularBuffer=on
  Delay2 : Delay  DelayLength=100  InitialCondition=0  UseCircularBuffer=on
  Gain : Gain  Gain=0.7
  Gain1 : Gain  Gain=0.5
  HDL Counter1 : hdlsllib/Sources/HDL Counter  CountType=Count limited  CountInit=0  CountStep=1  CountMax=1152  CountFromType=Initial value  CountFrom=0  CountResetPort=on  CountLoadPort=off  CountEnbPort=on  CountDirPort=off  CountDataType=Unsigned  CountWordLen=11  CountFracLen=0  CountSampTime=1
      settings: SourceProductBaseCode=HD
  Logical Operator1 : Logic  IconShape=distinctive  AllPortsSameDT=off  OutDataTypeStr=boolean
  Logical Operator2 : Logic  Operator=NOT  IconShape=distinctive  AllPortsSameDT=off  OutDataTypeStr=boolean
  Logical Operator3 : Logic  Inputs=3  IconShape=distinctive  AllPortsSameDT=off  OutDataTypeStr=boolean
  Relational Operator1 : RelationalOperator  Operator=>  OutDataTypeStr=boolean  RndMeth=Nearest
  Relational Operator2 : RelationalOperator  Operator=>  OutDataTypeStr=boolean  RndMeth=Nearest
  Relational Operator3 : RelationalOperator  OutDataTypeStr=boolean  RndMeth=Nearest
  Relational Operator4 : RelationalOperator  Operator=<=  OutDataTypeStr=boolean  RndMeth=Nearest
  Задержка максимального значения : Subsystem
  MiddleRdEn : Outport
  wires:
  MagMax/1 -> Gain/1
  Gain/1 -> Relational Operator1/2
  Logical Operator1/1 -> Delay2/1, Logical Operator2/1, HDL Counter1/2
  Relational Operator1/1 -> Logical Operator1/2
  Logical Operator2/1 -> HDL Counter1/1
  Constant/1 -> Relational Operator2/2
  Relational Operator2/1 -> Logical Operator1/1
  MagIn/1 -> Relational Operator1/1, Relational Operator2/1
  HDL Counter1/1 -> Delay1/1, Задержка максимального значения/1(AmpIn)
  Relational Operator3/1 -> Logical Operator3/1
  Relational Operator4/1 -> Logical Operator3/2
  Logical Operator3/1 -> MiddleRdEn/1
  Gain1/1 -> Add1/1, Add/1
  Constant3/1 -> Add/2, Add1/2
  "Reset "/1 -> Задержка максимального значения/2("Reset ")
  Задержка максимального значения/1(Out1) -> Gain1/1
  Delay1/1 -> Relational Operator4/1, Relational Operator3/1
  Add1/1 -> Relational Operator3/2
  Add/1 -> Relational Operator4/2
  Delay2/1 -> Logical Operator3/3

== system OFDMTxRx2211221/LTE_Detector_HDL/Frequency_Estimation/Cyclic_Prefix_Correlator/Moving_Average ==
  note: Use a comb filter followed by an integrator
      | to implement an efficient 9-tab moving average.
  dataIn : Inport
  Add : Sum  Inputs=-+  AccumDataTypeStr=fixdt(1,27,23)
  Add1 : Sum  AccumDataTypeStr=fixdt(1,27,23)
  Delay1 : Delay  DelayLength=128  InitialCondition=0
  Delay10 : Delay  DelayLength=1  InitialCondition=0  UseCircularBuffer=on
  Delay3 : Delay  DelayLength=1  InitialCondition=0  UseCircularBuffer=on
  Delay6 : Delay  DelayLength=1  InitialCondition=0  UseCircularBuffer=on
  Gain : Gain  Gain=1/128  OutDataTypeStr=fixdt(1,24,23)
  dataOut : Outport
  wires:
  dataIn/1 -> Add/2, Delay1/1
  Delay1/1 -> Add/1
  Add1/1 -> Delay6/1
  Delay10/1 -> Add1/2
  Delay6/1 -> Gain/1, Add1/1
  Delay3/1 -> dataOut/1
  Gain/1 -> Delay3/1
  Add/1 -> Delay10/1

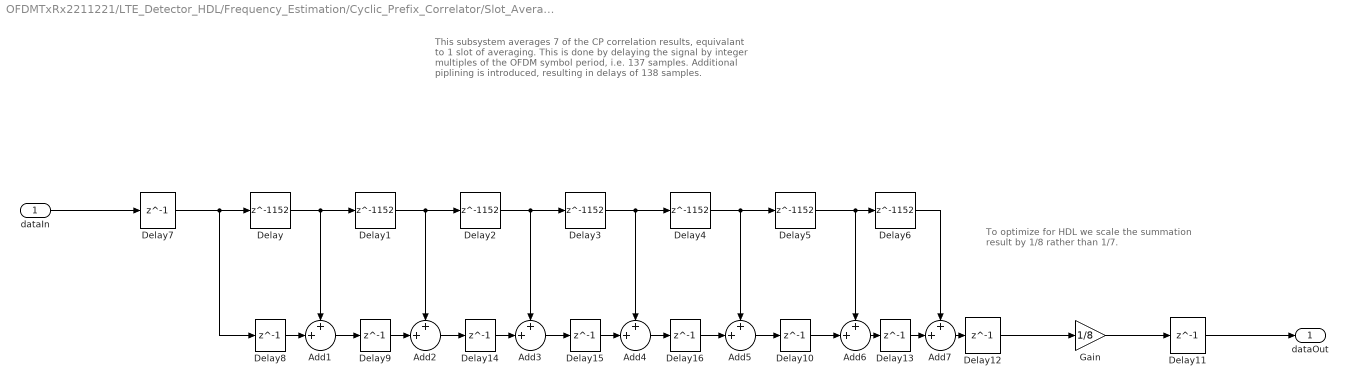
== system OFDMTxRx2211221/LTE_Detector_HDL/Frequency_Estimation/Cyclic_Prefix_Correlator/Slot_Average ==
  note: This subsystem averages 7 of the CP correlation results, equivalant to 1 slot of averaging. This is done by delaying the signal by integer multiples of the OFDM symbol period, i.e. 137 samples.
      |
      | Additional piplining is introduced, resulting in delays of 138 samples.
  note: To optimize for HDL we scale the summation result by 1/8 rather than 1/7.
  dataIn : Inport
  Add1 : Sum  Inputs=++|  AccumDataTypeStr=fixdt(1,28,23)
  Add2 : Sum  Inputs=++|  AccumDataTypeStr=fixdt(1,29,23)
  Add3 : Sum  Inputs=++|  OutDataTypeStr=fixdt(1,29,23)
  Add4 : Sum  Inputs=++|  AccumDataTypeStr=fixdt(1,29,23)
  Add5 : Sum  Inputs=++|  AccumDataTypeStr=fixdt(1,30,23)
  Add6 : Sum  Inputs=++|  AccumDataTypeStr=fixdt(1,30,23)
  Add7 : Sum  Inputs=++|  AccumDataTypeStr=fixdt(1,30,23)
  Delay{,1..6} (7 alike) : Delay  DelayLength=1152  InitialCondition=0
  Delay{7..16} (10 alike) : Delay  DelayLength=1  InitialCondition=0  UseCircularBuffer=on
  Gain : Gain  Gain=1/8  OutDataTypeStr=fixdt(1,24,23)
  dataOut : Outport
  wires:
  Delay4/1 -> Delay5/1, Add5/1
  Delay/1 -> Delay1/1, Add1/1
  Add1/1 -> Delay9/1
  Delay1/1 -> Delay2/1, Add2/1
  Delay3/1 -> Delay4/1, Add4/1
  Delay2/1 -> Delay3/1, Add3/1
  dataIn/1 -> Delay7/1
  Add2/1 -> Delay14/1
  Add3/1 -> Delay15/1
  Add4/1 -> Delay16/1
  Add5/1 -> Delay10/1
  Delay5/1 -> Add6/1, Delay6/1
  Delay7/1 -> Delay8/1, Delay/1
  Delay8/1 -> Add1/2
  Delay9/1 -> Add2/2
  Delay14/1 -> Add3/2
  Delay15/1 -> Add4/2
  Delay16/1 -> Add5/2
  Delay10/1 -> Add6/2
  Delay12/1 -> Gain/1
  Gain/1 -> Delay11/1
  Delay11/1 -> dataOut/1
  Delay6/1 -> Add7/1
  Add7/1 -> Delay12/1
  Add6/1 -> Delay13/1
  Delay13/1 -> Add7/2

== system OFDMTxRx2211221/LTE_Detector_HDL/Frequency_Estimation1/Angle_at_Maximum/Subsystem ==
  Amp : Inport
  MaxAmp : Inport  Port=2
  Compare To Constant : simulink/Logic and Bit Operations/Compare To Constant  relop===  const=7  OutDataTypeStr=boolean
  Constant : Constant  Value=6*10^-3
  Constant1 : Constant  Value=36
  Constant2 : Constant  Value=43
  Gain : Gain  Gain=0.7
  HDL Counter1 : hdlsllib/Sources/HDL Counter  CountType=Count limited  CountInit=0  CountStep=1  CountMax=1152  CountFromType=Initial value  CountFrom=0  CountResetPort=on  CountLoadPort=off  CountEnbPort=on  CountDirPort=off  CountDataType=Unsigned  CountWordLen=11  CountFracLen=0  CountSampTime=1
      settings: SourceProductBaseCode=HD
  HDL Counter2 : hdlsllib/Sources/HDL Counter  CountType=Count limited  CountInit=0  CountStep=1  CountMax=7  CountFromType=Initial value  CountFrom=0  CountResetPort=on  CountLoadPort=off  CountEnbPort=on  CountDirPort=off  CountDataType=Unsigned  CountWordLen=3  CountFracLen=0  CountSampTime=1
      settings: SourceProductBaseCode=HD
  Logical Operator1 : Logic  IconShape=distinctive  AllPortsSameDT=off  OutDataTypeStr=boolean
  Logical Operator2 : Logic  Operator=NOT  IconShape=distinctive  AllPortsSameDT=off  OutDataTypeStr=boolean
  Logical Operator3 : Logic  IconShape=distinctive  AllPortsSameDT=off  OutDataTypeStr=boolean
  Logical Operator4 : Logic  Operator=NOT  IconShape=distinctive  AllPortsSameDT=off  OutDataTypeStr=boolean
  Relational Operator1 : RelationalOperator  Operator=>  OutDataTypeStr=boolean  RndMeth=Nearest
  Relational Operator2 : RelationalOperator  Operator=>  OutDataTypeStr=boolean  RndMeth=Nearest
  Relational Operator3 : RelationalOperator  OutDataTypeStr=boolean  RndMeth=Nearest
  Relational Operator4 : RelationalOperator  Operator=<=  OutDataTypeStr=boolean  RndMeth=Nearest
  Window : Outport
  LastSampOfWindow : Outport  Port=2
  wires:
  MaxAmp/1 -> Gain/1
  Gain/1 -> Relational Operator1/2
  Logical Operator1/1 -> Logical Operator2/1, HDL Counter1/2
  Relational Operator1/1 -> Logical Operator1/2
  Logical Operator2/1 -> HDL Counter1/1
  Constant/1 -> Relational Operator2/2
  Relational Operator2/1 -> Logical Operator1/1
  Constant1/1 -> Relational Operator3/2
  Amp/1 -> Relational Operator2/1, Relational Operator1/1
  HDL Counter1/1 -> Relational Operator4/1, Relational Operator3/1
  Relational Operator3/1 -> Logical Operator3/1
  Constant2/1 -> Relational Operator4/2
  Relational Operator4/1 -> Logical Operator3/2
  Logical Operator3/1 -> HDL Counter2/2, Logical Operator4/1, Window/1
  Logical Operator4/1 -> HDL Counter2/1
  HDL Counter2/1 -> Compare To Constant/1
  Compare To Constant/1 -> LastSampOfWindow/1

== system OFDMTxRx2211221/LTE_Detector_HDL/Frequency_Estimation1/Angle_at_Maximum/Средняя сумма 8 текущих отсчетов ==
  note: Интегратор в окне для 8 отсчетов
  dataIn : Inport
  Add1 : Sum  AccumDataTypeStr=fixdt(1,27,23)
  Add2 : Sum  Inputs=-+  AccumDataTypeStr=fixdt(1,27,23)
  Delay1 : Delay  DelayLength=9  InitialCondition=0
  Delay2 : Delay  DelayLength=1  InitialCondition=0  UseCircularBuffer=on
  Gain : Gain  Gain=1/8  OutDataTypeStr=fixdt(1,24,23)
  dataOut : Outport
  wires:
  Delay1/1 -> Add2/1
  Add1/1 -> Delay2/1
  dataIn/1 -> Delay1/1, Add2/2
  Delay2/1 -> Gain/1, Add1/1
  Gain/1 -> dataOut/1
  Add2/1 -> Add1/2

== system OFDMTxRx2211221/LTE_Detector_HDL/Frequency_Estimation1/Angle_at_Maximum1/Subsystem ==
  Amp : Inport
  MaxAmp : Inport  Port=2
  Constant : Constant  Value=6*10^-3
  Constant1 : Constant  Value=60
  Constant2 : Constant  Value=67
  Gain : Gain  Gain=0.7
  HDL Counter1 : hdlsllib/Sources/HDL Counter  CountType=Count limited  CountInit=0  CountStep=1  CountMax=1152  CountFromType=Initial value  CountFrom=0  CountResetPort=on  CountLoadPort=off  CountEnbPort=on  CountDirPort=off  CountDataType=Unsigned  CountWordLen=11  CountFracLen=0  CountSampTime=1
      settings: SourceProductBaseCode=HD
  HDL Counter2 : hdlsllib/Sources/HDL Counter  CountType=Count limited  CountInit=0  CountStep=1  CountMax=7  CountFromType=Initial value  CountFrom=0  CountResetPort=on  CountLoadPort=off  CountEnbPort=on  CountDirPort=off  CountDataType=Unsigned  CountWordLen=3  CountFracLen=0  CountSampTime=1
      settings: SourceProductBaseCode=HD
  Logical Operator1 : Logic  IconShape=distinctive  AllPortsSameDT=off  OutDataTypeStr=boolean
  Logical Operator2 : Logic  Operator=NOT  IconShape=distinctive  AllPortsSameDT=off  OutDataTypeStr=boolean
  Logical Operator3 : Logic  IconShape=distinctive  AllPortsSameDT=off  OutDataTypeStr=boolean
  Logical Operator4 : Logic  Operator=NOT  IconShape=distinctive  AllPortsSameDT=off  OutDataTypeStr=boolean
  Relational Operator1 : RelationalOperator  Operator=>  OutDataTypeStr=boolean  RndMeth=Nearest
  Relational Operator2 : RelationalOperator  Operator=>  OutDataTypeStr=boolean  RndMeth=Nearest
  Relational Operator3 : RelationalOperator  OutDataTypeStr=boolean  RndMeth=Nearest
  Relational Operator4 : RelationalOperator  Operator=<=  OutDataTypeStr=boolean  RndMeth=Nearest
  Window : Outport
  LastSampOfWindow : Outport  Port=2
  wires:
  MaxAmp/1 -> Gain/1
  Gain/1 -> Relational Operator1/2
  Logical Operator1/1 -> Logical Operator2/1, HDL Counter1/2
  Relational Operator1/1 -> Logical Operator1/2
  Logical Operator2/1 -> HDL Counter1/1
  Constant/1 -> Relational Operator2/2
  Relational Operator2/1 -> Logical Operator1/1
  Constant1/1 -> Relational Operator3/2
  Amp/1 -> Relational Operator2/1, Relational Operator1/1
  HDL Counter1/1 -> Relational Operator4/1, Relational Operator3/1
  Relational Operator3/1 -> Logical Operator3/1
  Constant2/1 -> Relational Operator4/2
  Relational Operator4/1 -> Logical Operator3/2
  Logical Operator3/1 -> HDL Counter2/2, Logical Operator4/1, Window/1
  Logical Operator4/1 -> HDL Counter2/1
  HDL Counter2/1 -> LastSampOfWindow/1

== system OFDMTxRx2211221/LTE_Detector_HDL/Frequency_Estimation1/Cyclic_Prefix_Correlator/Moving_Average ==
  note: Интегратор в окне для 64 отсчетов
  dataIn : Inport
  Add1 : Sum  AccumDataTypeStr=fixdt(1,27,23)
  Add2 : Sum  Inputs=-+  AccumDataTypeStr=fixdt(1,27,23)
  Delay1 : Delay  DelayLength=64  InitialCondition=0
  Delay2 : Delay  DelayLength=1  InitialCondition=0  UseCircularBuffer=on
  Delay3 : Delay  DelayLength=1  InitialCondition=0  UseCircularBuffer=on
  Gain : Gain  Gain=1/64  OutDataTypeStr=fixdt(1,24,23)
  Scope14 : Scope  NumInputPorts=3
  dataOut : Outport
  wires:
  Delay1/1 -> Add2/1
  Add1/1 -> Delay2/1
  dataIn/1 -> Delay1/1, Add2/2
  Delay2/1 -> Gain/1, Add1/1
  Delay3/1 -> dataOut/1
  Gain/1 -> Delay3/1
  Add2/1 -> Add1/2

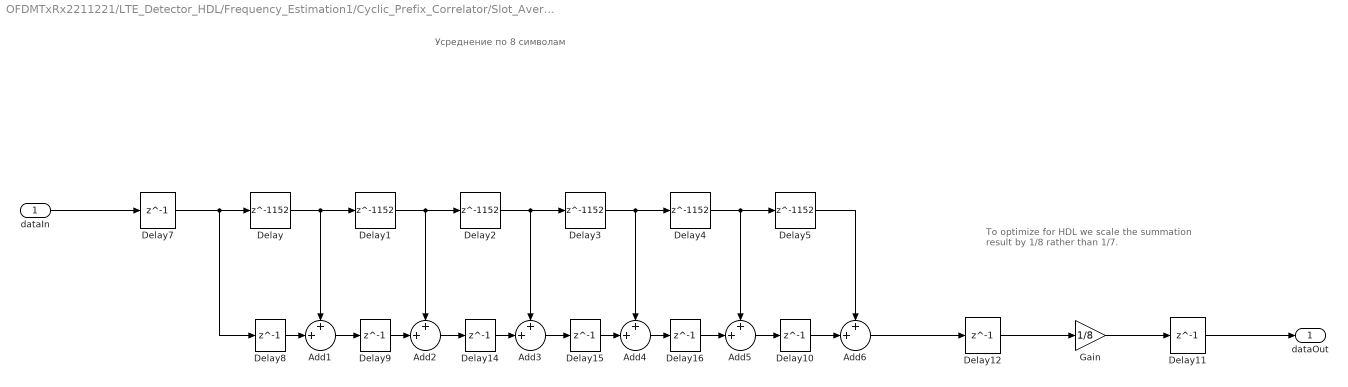
== system OFDMTxRx2211221/LTE_Detector_HDL/Frequency_Estimation1/Cyclic_Prefix_Correlator/Slot_Average ==
  note: Усреднение по 8 символам
  note: To optimize for HDL we scale the summation result by 1/8 rather than 1/7.
  dataIn : Inport
  Add1 : Sum  Inputs=++|  AccumDataTypeStr=fixdt(1,28,23)
  Add2 : Sum  Inputs=++|  AccumDataTypeStr=fixdt(1,29,23)
  Add3 : Sum  Inputs=++|  OutDataTypeStr=fixdt(1,29,23)
  Add4 : Sum  Inputs=++|  AccumDataTypeStr=fixdt(1,29,23)
  Add5 : Sum  Inputs=++|  AccumDataTypeStr=fixdt(1,30,23)
  Add6 : Sum  Inputs=++|  AccumDataTypeStr=fixdt(1,30,23)
  Delay{,1..5} (6 alike) : Delay  DelayLength=1152  InitialCondition=0
  Delay{7..12,14..16} (9 alike) : Delay  DelayLength=1  InitialCondition=0  UseCircularBuffer=on
  Gain : Gain  Gain=1/8  OutDataTypeStr=fixdt(1,24,23)
  dataOut : Outport
  wires:
  Delay4/1 -> Delay5/1, Add5/1
  Delay/1 -> Delay1/1, Add1/1
  Add1/1 -> Delay9/1
  Delay1/1 -> Delay2/1, Add2/1
  Delay3/1 -> Delay4/1, Add4/1
  Delay2/1 -> Delay3/1, Add3/1
  dataIn/1 -> Delay7/1
  Add2/1 -> Delay14/1
  Add3/1 -> Delay15/1
  Add4/1 -> Delay16/1
  Add5/1 -> Delay10/1
  Delay5/1 -> Add6/1
  Add6/1 -> Delay12/1
  Delay7/1 -> Delay8/1, Delay/1
  Delay8/1 -> Add1/2
  Delay9/1 -> Add2/2
  Delay14/1 -> Add3/2
  Delay15/1 -> Add4/2
  Delay16/1 -> Add5/2
  Delay10/1 -> Add6/2
  Delay12/1 -> Gain/1
  Gain/1 -> Delay11/1
  Delay11/1 -> dataOut/1

== system OFDMTxRx2211221/LTE_Detector_HDL/Frequency_Estimation2/Cyclic_Prefix_Correlator/Moving_Average ==
  note: Use a comb filter followed by an integrator
      | to implement an efficient 9-tab moving average.
  dataIn : Inport
  Add : Sum  Inputs=-+  AccumDataTypeStr=fixdt(1,27,23)
  Add1 : Sum  AccumDataTypeStr=fixdt(1,27,23)
  Delay1 : Delay  DelayLength=128  InitialCondition=0
  Delay10 : Delay  DelayLength=1  InitialCondition=0  UseCircularBuffer=on
  Delay2 : Delay  DelayLength=1  InitialCondition=0  UseCircularBuffer=on
  Delay3 : Delay  DelayLength=1  InitialCondition=0  UseCircularBuffer=on
  Gain : Gain  Gain=1/128  OutDataTypeStr=fixdt(1,24,23)
  dataOut : Outport
  wires:
  Add/1 -> Delay10/1
  dataIn/1 -> Add/2, Delay1/1
  Delay1/1 -> Add/1
  Add1/1 -> Delay2/1
  Delay10/1 -> Add1/2
  Delay2/1 -> Gain/1, Add1/1
  Gain/1 -> Delay3/1
  Delay3/1 -> dataOut/1

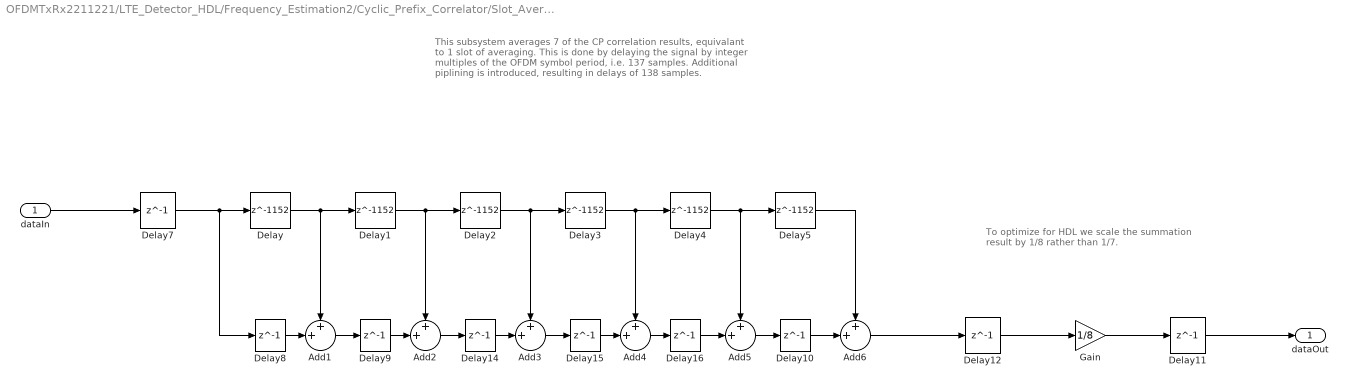
== system OFDMTxRx2211221/LTE_Detector_HDL/Frequency_Estimation2/Cyclic_Prefix_Correlator/Slot_Average ==
  note: This subsystem averages 7 of the CP correlation results, equivalant to 1 slot of averaging. This is done by delaying the signal by integer multiples of the OFDM symbol period, i.e. 137 samples.
      |
      | Additional piplining is introduced, resulting in delays of 138 samples.
  note: To optimize for HDL we scale the summation result by 1/8 rather than 1/7.
  dataIn : Inport
  Add1 : Sum  Inputs=++|  AccumDataTypeStr=fixdt(1,28,23)
  Add2 : Sum  Inputs=++|  AccumDataTypeStr=fixdt(1,29,23)
  Add3 : Sum  Inputs=++|  OutDataTypeStr=fixdt(1,29,23)
  Add4 : Sum  Inputs=++|  AccumDataTypeStr=fixdt(1,29,23)
  Add5 : Sum  Inputs=++|  AccumDataTypeStr=fixdt(1,30,23)
  Add6 : Sum  Inputs=++|  AccumDataTypeStr=fixdt(1,30,23)
  Delay{,1..5} (6 alike) : Delay  DelayLength=1152  InitialCondition=0
  Delay{7..12,14..16} (9 alike) : Delay  DelayLength=1  InitialCondition=0  UseCircularBuffer=on
  Gain : Gain  Gain=1/8  OutDataTypeStr=fixdt(1,24,23)
  dataOut : Outport
  wires:
  Delay4/1 -> Delay5/1, Add5/1
  Delay/1 -> Delay1/1, Add1/1
  Add1/1 -> Delay9/1
  Delay1/1 -> Delay2/1, Add2/1
  Delay3/1 -> Delay4/1, Add4/1
  Delay2/1 -> Delay3/1, Add3/1
  dataIn/1 -> Delay7/1
  Add2/1 -> Delay14/1
  Add3/1 -> Delay15/1
  Add4/1 -> Delay16/1
  Add5/1 -> Delay10/1
  Delay5/1 -> Add6/1
  Add6/1 -> Delay12/1
  Delay7/1 -> Delay8/1, Delay/1
  Delay8/1 -> Add1/2
  Delay9/1 -> Add2/2
  Delay14/1 -> Add3/2
  Delay15/1 -> Add4/2
  Delay16/1 -> Add5/2
  Delay10/1 -> Add6/2
  Delay12/1 -> Gain/1
  Gain/1 -> Delay11/1
  Delay11/1 -> dataOut/1

== system OFDMTxRx2211221/LTE_Detector_HDL/Эквалайзинг забита только формула/Subsystem/2interp ==
  y1 : Inport
  y2 : Inport  Port=2
  y3 : Inport  Port=3
  Constant2 : Constant
  Constant3 : Constant  Value=11
  Constant4 : Constant  Value=21
  "KoefA " : Subsystem
  Subsystem : Subsystem
  Subsystem1 : Subsystem
  a : Outport
  b : Outport  Port=2
  c : Outport  Port=3
  wires:
  y1/1 -> Subsystem1/1(y1), Subsystem/1(y1), "KoefA "/1(y1)
  y2/1 -> Subsystem/2("y2 "), "KoefA "/2(y2)
  y3/1 -> "KoefA "/3(y3)
  Constant2/1 -> "KoefA "/4(x1), Subsystem1/4(x1), Subsystem/4(x1)
  Constant3/1 -> "KoefA "/5(x2), Subsystem/5("x2 ")
  Constant4/1 -> "KoefA "/6(x3)
  "KoefA "/1(Out1) -> a/1, Subsystem1/2(a), Subsystem/3(a)
  Subsystem/1(b) -> Subsystem1/3(b), b/1
  Subsystem1/1(c) -> c/1

== system OFDMTxRx2211221/LTE_Detector_HDL/Frequency_Estimation/Angle_at_Maximum/Нахождение окрестности середины ЗИ/Задержка максимального значения ==
  AmpIn : Inport
  "Reset " : Inport  Port=2
  Logical Operator : Logic  Operator=OR  IconShape=distinctive  AllPortsSameDT=off  OutDataTypeStr=boolean
  Relational Operator : RelationalOperator  Operator=>  OutDataTypeStr=boolean  RndMeth=Nearest
  Unit Delay Enabled : simulink_need_slupdate/Unit Delay Enabled  vinit=0.0  tsamp=-1
      settings: SourceProductName=Simulink  SourceProductBaseCode=SL
  Out1 : Outport
  wires:
  Logical Operator/1 -> Unit Delay Enabled/2
  Unit Delay Enabled/1 -> Out1/1, Relational Operator/2
  Relational Operator/1 -> Logical Operator/1
  "Reset "/1 -> Logical Operator/2
  AmpIn/1 -> Relational Operator/1, Unit Delay Enabled/1
